simulink model "Sub4"  (R2024a)
settings: Solver=FixedStepDiscrete  StartTime=0.0  StopTime=4.5  FixedStep=75e-6  RelTol=1e-3  EnableMultiTasking=on
undefined symbols (not defined in the file or in its folder): D1, D11, Delta
libraries: spsSeriesRLCBranchLib x41, spsLoadFlowBusLib x29, spsDistributedParametersLineLib x19, spsThreePhaseSeriesRLCLoadLib x15, spsThreePhaseTransformerTwoWindingsLib x13, spsThreePhaseParallelRLCLoadLib x11, spsThreePhaseVIMeasurementLib x11, spsSynchronousMachinepuStandardLib x7, spsExcitationSystemLib x7, spsHydraulicTurbineandGovernorLib x7, spsGenericPowerSystemStabilizerLib x7, spsMultiBandPowerSystemStabilizerLib x7
(part 3 of 5)

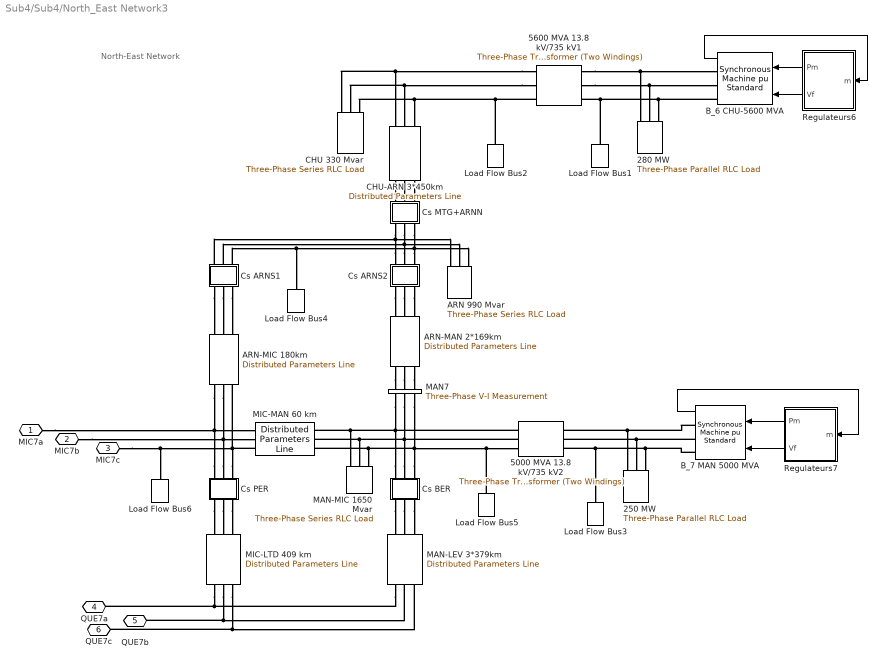
== system Sub4/Sub4/North_East Network3 ==
  note: North-East Network
  250 MW : spsThreePhaseParallelRLCLoadLib/Three-Phase Parallel RLC Load  LConnTagsString=A|B|C  Configuration=Y (grounded)  NominalVoltage=(13800)*1  Vabc=[1e3 1e3 1e3]  Vabcp=[1e3 1e3 1e3]  NominalFrequency=60  UnbalancedPower=off  ActivePower=250000000  InductivePower=0  CapacitivePower=0  Pabc=[10e3 9e3 11e3]  QLabc=[100 90 110]  QCabc=[100 90 110]  Pabcp=[10e3 9e3 11e3]  QLabcp=[100 90 110]  QCabcp=[100 90 110]  Measurements=None  LoadType=constant PQ
  280 MW : spsThreePhaseParallelRLCLoadLib/Three-Phase Parallel RLC Load  LConnTagsString=A|B|C  Configuration=Y (grounded)  NominalVoltage=(13800)*1  Vabc=[1e3 1e3 1e3]  Vabcp=[1e3 1e3 1e3]  NominalFrequency=60  UnbalancedPower=off  ActivePower=280000000  InductivePower=0  CapacitivePower=0  Pabc=[10e3 9e3 11e3]  QLabc=[100 90 110]  QCabc=[100 90 110]  Pabcp=[10e3 9e3 11e3]  QLabcp=[100 90 110]  QCabcp=[100 90 110]  Measurements=None  LoadType=constant PQ
  5000 MVA 13.8 kV/735 kV2 : spsThreePhaseTransformerTwoWindingsLib/Three-Phase Transformer (Two Windings)  Winding1Connection=Delta (D1)  Winding2Connection=Yg  CoreType=Three single-phase transformers  SetSaturation=off  Hysteresis=off  DataFile='basic_model'  SetInitialFlux=off  Measurements=None  UNITS=pu  NominalPower=[ 5000e6 60 ]  Winding1="[ 13.8e3 0.002  0.0]"  Winding2=[ 735e3 0.002 0.12]  Rm=500  Lm=500  L0=0.5  Saturation="[ 0,0  ;  0.005,1.2  ;  1.0,1.4 ]"  InitialFluxes=[ 0.8 , -0.8 , 0.7 ]  BreakLoop=off  DiscreteSolver=Trapezoidal iterative  DataType=off  TransfoNumber=0
  5600 MVA 13.8 kV/735 kV1 : spsThreePhaseTransformerTwoWindingsLib/Three-Phase Transformer (Two Windings)  Winding1Connection=Delta (D1)  Winding2Connection=Yg  CoreType=Three single-phase transformers  SetSaturation=off  Hysteresis=off  DataFile='basic_model'  SetInitialFlux=off  Measurements=None  UNITS=pu  NominalPower=[ 5600e6 60 ]  Winding1="[ 13.8e3 0.002  0.0]"  Winding2=[ 735e3 0.002 0.12]  Rm=500  Lm=500  L0=0.5  Saturation="[ 0,0  ;  0.005,1.2  ;  1.0,1.4 ]"  InitialFluxes=[ 0.8 , -0.8 , 0.7 ]  BreakLoop=off  DiscreteSolver=Trapezoidal iterative  DataType=off  TransfoNumber=0
  ARN 990 Mvar : spsThreePhaseSeriesRLCLoadLib/Three-Phase Series RLC Load  LConnTagsString=A|B|C  Configuration=Y (grounded)  NominalVoltage=735e3  Vabc=[1e3 1e3 1e3]  Vabcp=[1e3 1e3 1e3]  NominalFrequency=60  UnbalancedPower=off  ActivePower=3300000  InductivePower=990e6  CapacitivePower=0  Pabc=[10e3 9e3 11e3]  QLabc=[100 90 110]  QCabc=[100 90 110]  Pabcp=[10e3 9e3 11e3]  QLabcp=[100 90 110]  QCabcp=[100 90 110]  Measurements=None  LoadType=constant Z
  ARN-MAN 2*169km : spsDistributedParametersLineLib/Distributed Parameters Line  Phases=3  Length=169  Frequency=60  Resistance="[0.01273  0.3864]/2"  Inductance="[0.9337e-3  4.1264e-3]/2"  Capacitance=[12.74e-9 7.751e-9]*2  x1=[-0.000975 1.66426565004939e-09 276427.296115043 -784420.047795663;-0.0009 1.59178701377787e-09 298492.841238135 -776291.834335438;-0.000825 1.51803592732269e-09 320319.775751036 -767543.065060509;-0.00075 1.44307134617394e-09 341890.651536257 -758180.733603173;-0.000675 1.36695319587079e-09 363188.225165743 -748212.324067948;-0.0006 1.28974232409794e-09 384195.471684998 -737645.805048896;-0.000525 1.21150045204493e-09 404895.598222576 -726489.623259648;-0.00045 1.13229012506714e-09 425272.057414045 -714752.696781229;-0.000375 1.05217466268798e-09 445308.560629698 -702444.407933087;-0.0003 9.71218107982286e-10 464989.090995432 -689574.595773002;-0.000225 8.89485176381205e-10 484297.916196397 -676153.548231903;-0.00015 8.07041203939704e-10 503219.601053161 -662191.993889842;-7.5e-05 7.23952095107918e-10 521739.019860361 -647701.093399743]  x2=[-0.000975 1.50301647460342e-09 170603.864508789 -782532.609847258;-0.0009 1.45617880236044e-09 192658.333570876 -777396.800423983;-0.000825 1.40817708306313e-09 214558.794508878 -771639.551893019;-0.00075 1.35904968855145e-09 236287.740429409 -765265.466510753;-0.000675 1.3088358905129e-09 257827.801545564 -758279.639623513;-0.0006 1.25757582908933e-09 279161.759062062 -750687.655594424;-0.000525 1.20531048078955e-09 300272.558939683 -742495.583339361;-0.00045 1.15208162573329e-09 321143.325528012 -733709.971475538;-0.000375 1.09793181425286e-09 341757.375055572 -724337.843086658;-0.0003 1.04290433287904e-09 362098.228966576 -714386.690108754;-0.000225 9.87043169738486e-10 382149.627093632 -703864.467341261;-0.00015 9.30392979390309e-10 401895.540655875 -692779.586088062;-7.5e-05 8.72999047129898e-10 421320.185072126 -681140.907433628]  x3=[-0.000975 -6.52958955805801e-13 1329.1720136715 -2414.87241463394;-0.0009 -8.44230426340621e-13 1396.90953145447 -2376.33167069261;-0.000825 -1.03482703198978e-12 1463.53038113142 -2335.89132357282;-0.00075 -1.22459641274296e-12 1528.98130701446 -2293.5837006693;-0.000675 -1.41338686986074e-12 1593.20998863487 -2249.44262204848;-0.0006 -1.6010474871403e-12 1656.1650825673 -2203.50337341321;-0.000525 -1.78742825155548e-12 1717.7962634729 -2155.80267789598;-0.00045 -1.97238017317495e-12 1778.05426432864 -2106.37866670291;-0.000375 -2.1557554042624e-12 1836.89091581062 -2055.27084863236;-0.0003 -2.33740735746385e-12 1894.25918479988 -2002.52007849212;-0.000225 -2.51719082298728e-12 1950.11321197994 -1948.16852444071;-0.00015 -2.69496208468112e-12 2004.40834849608 -1892.25963427884;-7.5e-05 -2.87057903491877e-12 2057.10119164691 -1834.83810071787]  x4=[-0.000975 1.02278224953366e-11 681.724417840483 -9455.17189861565;-0.0009 9.98598605323801e-12 948.756484621656 -9432.11979189438;-0.000825 9.73616696667912e-12 1215.03012998548 -9401.52779292775;-0.00075 9.47856493721543e-12 1480.33249885398 -9363.42035649164;-0.000675 9.21338588796783e-12 1744.45151257275 -9317.8279450877;-0.0006 8.94084179901093e-12 2007.17603844337 -9264.787004592;-0.000525 8.66115053791936e-12 2268.29605849967 -9204.33993512082;-0.00045 8.37453568560783e-12 2527.60283739291 -9136.53505713663;-0.000375 8.08122635760391e-12 2784.88908925156 -9061.42657282144;-0.0003 7.78145702089663e-12 3039.94914338249 -8979.07452274841;-0.000225 7.47546730650714e-12 3292.57910868098 -8889.54473788635;-0.00015 7.1635018179313e-12 3542.57703661814 -8792.90878697541;-7.5e-05 6.84580993560747e-12 3789.74308267548 -8689.24391931618]  x5=0.000955765248222805  V1=ones(3,3)  V2=ones(3,3)  I1=ones(3,3)  I2=ones(3,3)  nHarmo=1  Measurements=None  Decoupling=on  VsMag0=[679080.965035306 679082.342856188 679080.506296934]  VrMag0=[653943.402704951 653944.061381449 653943.214719902]  VsAngle0=[10.4723030523782 -109.527808757273 130.472146471772]  VrAngle0=[3.35889302260268 -116.641159314998 123.358816875039]  IsMag0=[2259.59659727747 2259.62910081935 2259.62302793109]  IrMag0=[7771.00845150682 7771.0004925988 7770.97273571783]  IsAngle0=[19.8888438810371 -100.110858095183 139.888279140977]  IrAngle0=[-4.81594167233342 -124.816211863633 115.183974051701]
      settings: AttributesFormatString=\n  LibrarySourceBlock=sps_lib/Power Grid Elements/Distributed Parameters Line
  ARN-MIC 180km : spsDistributedParametersLineLib/Distributed Parameters Line  Phases=3  Length=180  Frequency=60  Resistance="[0.01273  0.3864]"  Inductance="[0.9337e-3  4.1264e-3]"  Capacitance=[12.74e-9 7.751e-9]  x1=[-0.00105 1.25846980374652e-09 262529.955827328 -774207.772445671;-0.000975 1.18990309098791e-09 284312.34957459 -766476.523484284;-0.0009 1.12038518790449e-09 305867.468379727 -758132.564917507;-0.000825 1.04997166604432e-09 327178.08141057 -749182.566778153;-0.00075 9.78718812899427e-10 348227.153289126 -739633.683557793;-0.000675 9.066835869104e-10 368997.857709397 -729493.548487572;-0.0006 8.33923571934722e-10 389473.590888071 -718770.267436316;-0.000525 7.60496931215097e-10 409637.984837336 -707472.412430826;-0.00045 6.86462360884652e-10 429474.920449193 -695609.014803529;-0.000375 6.11879043046142e-10 448968.540380829 -683189.557972972;-0.0003 5.36806598462684e-10 468103.261730734 -670223.969862923;-0.000225 4.61305038897832e-10 486863.788495431 -656722.614966137;-0.00015 3.85434719143088e-10 505235.123796871 -642696.286059139;-7.5e-05 3.09256288771211e-10 523202.581870704 -628156.195574648]  x2=[-0.00105 4.56021511773203e-09 126759.491965578 -811882.989724351;-0.000975 4.50169247794927e-09 149661.239004126 -807974.954383031;-0.0009 4.43957125407784e-09 172443.349138107 -803421.036225608;-0.000825 4.37390110487363e-09 195087.610697259 -798224.875584581;-0.00075 4.3047345260491e-09 217575.92220536 -792390.626191262;-0.000675 4.23212680830911e-09 239890.306850274 -785922.951855348;-0.0006 4.15613599315226e-09 262012.926854336 -778827.022736746;-0.000525 4.07682282647349e-09 283926.097733603 -771108.511212621;-0.00045 3.99425071000473e-09 305612.302434556 -762773.587342989;-0.000375 3.90848565063247e-09 327054.205336969 -753828.913938461;-0.0003 3.81959620763294e-09 348234.666111732 -744281.641234101;-0.000225 3.7276534378668e-09 369136.753422575 -734139.401173629;-0.00015 3.63273083897744e-09 389743.758460713 -723410.301308568;-7.5e-05 3.53490429063805e-09 410039.208301618 -712102.91831719]  x3=[-0.00105 3.52588969292103e-12 -44.8517351585408 -825.879343626934;-0.000975 3.77869229184614e-12 -21.4861584038212 -826.817643960785;-0.0009 4.02847426196908e-12 1.89659405717708 -827.094998920788;-0.000825 4.27503593140473e-12 25.277830409905 -826.711186793632;-0.00075 4.51818020252705e-12 48.6388600517669 -825.666514392858;-0.000675 4.75771270952595e-12 71.961008533103 -823.9618168136;-0.0006 4.9934419737803e-12 95.2256324852582 -821.598456765019;-0.000525 5.22517955692303e-12 118.414134523806 -818.578323480979;-0.00045 5.45274021147589e-12 141.507978115012 -814.903831209816;-0.000375 5.67594202893342e-12 164.488702393657 -810.577917284431;-0.0003 5.89460658517784e-12 187.337936920371 -805.604039774227;-0.000225 6.10855908310858e-12 210.037416366677 -799.986174720782;-0.00015 6.31762849237237e-12 232.56899511602 -793.728812959465;-7.5e-05 6.52164768608231e-12 254.914661769092 -786.836956529525]  x4=[-0.00105 3.68388905079501e-12 787.856966725056 -5164.02437043881;-0.000975 3.27425714129396e-12 933.532622338121 -5139.68710729563;-0.0009 2.86200784073198e-12 1078.46202625642 -5111.24125691872;-0.000825 2.44747069489231e-12 1222.52932413195 -5078.70955848564;-0.00075 2.03097707842669e-12 1365.61935077109 -5042.11801733838;-0.000675 1.61285992995958e-12 1507.6177221959 -5001.49588419504;-0.0006 1.19345348594203e-12 1648.41092708092 -4956.87563176734;-0.000525 7.73093013468282e-13 1787.88641749236 -4908.29292880234;-0.00045 3.52114542268281e-13 1925.93269885724 -4855.78661156945;-0.000375 -6.91454039092747e-14 2062.43941909041 -4799.39865281531;-0.0003 -4.90350076308906e-13 2197.29745680833 -4739.17412821136;-0.000225 -9.11162770360144e-13 2330.39900855907 -4675.16118032112;-0.00015 -1.33124709483401e-12 2461.63767499866 -4607.41098011569;-7.5e-05 -1.75026724074904e-12 2590.90854594518 -4535.97768606851]  x5=0.00101797482059234  V1=ones(3,3)  V2=ones(3,3)  I1=ones(3,3)  I2=ones(3,3)  nHarmo=1  Measurements=None  Decoupling=on  VsMag0=[667492.500318997 667493.817536454 667492.030186196]  VrMag0=[670930.718084451 670931.402748886 670930.538861588]  VsAngle0=[11.4115363399382 -108.588575536837 131.411382483017]  VrAngle0=[1.55396261635725 -118.446088813397 121.553886266157]  IsMag0=[678.171382863534 678.181184845914 678.186053012205]  IrMag0=[4283.30300695155 4283.29854095558 4283.28683546946]  IsAngle0=[-10.4293295371599 -130.428376510184 109.570429816024]  IrAngle0=[1.35460954054385 -118.645605751902 121.354553630566]
      settings: AttributesFormatString=\n  LibrarySourceBlock=sps_lib/Power Grid Elements/Distributed Parameters Line
  "B_6 CHU-5600 MVA " : spsSynchronousMachinepuStandardLib/Synchronous Machine pu Standard  PresetModel=No  MechanicalLoad=Mechanical power Pm  ShowDetailedParameters=on  RotorType=Salient-pole  Units=per unit standard parameters  MeasurementBus=off  NominalParameters="[ 5600E6  13800   60 ]"  Reactances1=[ 31 32 33 34 35 36 37 ]  Reactances2=[ 1.305, 0.296, 0.252, 0.474, 0.243, 0.18 ]  dAxisTimeConstants=Short-circuit  qAxisTimeConstants=Open-circuit  TimeConstants1=[]  TimeConstants2=[]  TimeConstants3=[]  TimeConstants4=[]  TimeConstants5=[ 1.01, 0.053, 0.1 ]  TimeConstants6=[]  TimeConstants7=[]  TimeConstants8=[]  StatorResistance=2.8544e-3  Mechanical="[ 4.0 0  32]"  PolePairs=32  InitialConditions=[0 -61.7964 0.894782 0.894782 0.894782 8.48442 -111.516 128.484 1.31361]  SetSaturation=off  Saturation=[0.6404,0.7127,0.8441,0.9214,0.9956,1.082,1.19,1.316,1.457;0.7,0.7698,0.8872,0.9466,0.9969,1.046,1.1,1.151,1.201]  LoadFlowParameters=[1 5000000000 0 0 0]  TsPowergui=0  TsBlock=-1  IterativeModel=Trapezoidal non iterative  IterativeDiscreteModel=Trapezoidal non iterative  BusType=PV  Pref=5000000000  Qref=0  Qmin=-Inf  Qmax=Inf  PLF=0  QLF=0
  B_7 MAN 5000 MVA : spsSynchronousMachinepuStandardLib/Synchronous Machine pu Standard  PresetModel=No  MechanicalLoad=Mechanical power Pm  ShowDetailedParameters=on  RotorType=Salient-pole  Units=per unit standard parameters  MeasurementBus=off  NominalParameters="[ 5000E6  13800   60 ]"  Reactances1=[ 31 32 33 34 35 36 37 ]  Reactances2=[ 1.305, 0.296, 0.252, 0.474, 0.243, 0.18 ]  dAxisTimeConstants=Short-circuit  qAxisTimeConstants=Open-circuit  TimeConstants1=[]  TimeConstants2=[]  TimeConstants3=[]  TimeConstants4=[]  TimeConstants5=[ 1.01, 0.053, 0.1 ]  TimeConstants6=[]  TimeConstants7=[]  TimeConstants8=[]  StatorResistance=2.8544e-3  Mechanical="[ 3.7 0  32]"  PolePairs=32  InitialConditions=[0 -81.9543 0.907703 0.907703 0.907703 -8.76021 -128.76 111.24 1.25655]  SetSaturation=off  Saturation=[0.6404,0.7127,0.8441,0.9214,0.9956,1.082,1.19,1.316,1.457;0.7,0.7698,0.8872,0.9466,0.9969,1.046,1.1,1.151,1.201]  LoadFlowParameters=[1 4500000000 0 0 0]  TsPowergui=0  TsBlock=-1  IterativeModel=Trapezoidal non iterative  IterativeDiscreteModel=Trapezoidal non iterative  BusType=PV  Pref=4500000000  Qref=0  Qmin=-Inf  Qmax=Inf  PLF=0  QLF=0
  CHU 330 Mvar : spsThreePhaseSeriesRLCLoadLib/Three-Phase Series RLC Load  LConnTagsString=A|B|C  Configuration=Y (grounded)  NominalVoltage=735e3  Vabc=[1e3 1e3 1e3]  Vabcp=[1e3 1e3 1e3]  NominalFrequency=60  UnbalancedPower=off  ActivePower=1100000  InductivePower=330e6  CapacitivePower=0  Pabc=[10e3 9e3 11e3]  QLabc=[100 90 110]  QCabc=[100 90 110]  Pabcp=[10e3 9e3 11e3]  QLabcp=[100 90 110]  QCabcp=[100 90 110]  Measurements=None  LoadType=constant Z
  CHU-ARN 3*450km : spsDistributedParametersLineLib/Distributed Parameters Line  Phases=3  Length=450  Frequency=60  Resistance="[0.01273  0.3864]/3"  Inductance="[0.9337e-3  4.1264e-3]/3"  Capacitance=[12.74e-9 7.751e-9]*3  x1=[-0.00255 1.83974130674967e-09 0 0;-0.002475 1.75252338019027e-09 0 0;-0.0024 1.66390451325524e-09 0 0;-0.002325 1.57395554651092e-09 0 0;-0.00225 1.48274838378504e-09 0 0;-0.002175 1.39035593468798e-09 0 0;-0.0021 1.29685205632988e-09 0 0;-0.002025 1.20231149428046e-09 0 0;-0.00195 1.10680982281849e-09 0 0;-0.001875 1.01042338451892e-09 0 0;-0.0018 9.13229229225756e-10 0 0;-0.001725 8.15305052459629e-10 0 0;-0.00165 7.1672913330915e-10 0 0;-0.001575 6.17580271855829e-10 242668.42145696 -732167.508894537;-0.0015 5.17937726182481e-10 263270.288908628 -725014.590467308;-0.001425 4.17881149015535e-10 283661.702119514 -717282.106469554;-0.00135 3.17490524051862e-10 303826.360505894 -708976.238130673;-0.001275 2.1684610202103e-10 323748.144748385 -700103.62503473;-0.0012 1.160283365341e-10 343411.129677477 -690671.359812879;-0.001125 1.51178197702368e-11 362799.597003872 -680686.98247362;-0.00105 -8.58047819474405e-11 381898.047883441 -670158.474375432;-0.000975 -1.86658792635286e-10 400691.215306768 -659094.251846596;-0.0009 -2.87363591140274e-10 419164.076303361 -647503.159457315;-0.000825 -3.87838675587315e-10 437301.863950782 -635394.462949494;-0.00075 -4.88003727731222e-10 455090.079179103 -622777.841829852;-0.000675 -5.87778677161888e-10 472514.502361241 -609663.381632272;-0.0006 -6.87083765311346e-10 489561.204679905 -596061.565855578;-0.000525 -7.85839609211549e-10 506216.559262086 -581983.267583187;-0.00045 -8.83967264951897e-10 522467.252072166 -567439.740791332;-0.000375 -9.81388290785795e-10 538300.292554956 -552442.611352808;-0.0003 -1.07802480983578e-09 553703.024020149 -537003.867743423;-0.000225 -1.17379957234712e-09 568663.13375988 -521135.8514586;-0.00015 -1.26863601744006e-09 583168.662891321 -504851.247147766;-7.5e-05 -1.36245833431144e-09 597208.015916427 -488163.072474445]  x2=[-0.00255 2.68580757791396e-09 0 0;-0.002475 2.65982228221435e-09 0 0;-0.0024 2.63171076527898e-09 0 0;-0.002325 2.60149549902437e-09 0 0;-0.00225 2.56920063707206e-09 0 0;-0.002175 2.53485199544056e-09 0 0;-0.0021 2.49847703190844e-09 0 0;-0.002025 2.460104824065e-09 0 0;-0.00195 2.41976604606606e-09 0 0;-0.001875 2.37749294411356e-09 0 0;-0.0018 2.3333193106784e-09 0 0;-0.001725 2.28728045748726e-09 0 0;-0.00165 2.23941318729497e-09 0 0;-0.001575 2.18975576446493e-09 -54170.285736792 -807523.190587312;-0.0015 2.13834788438116e-09 -31319.4766467201 -808731.868853913;-0.001425 2.08523064171644e-09 -8443.63124622096 -809294.059238565;-0.00135 2.03044649758183e-09 14438.9638639046 -809209.312334876;-0.001275 1.97403924558393e-09 37310.0166872409 -808477.695888224;-0.0012 1.91605397681692e-09 60151.2444540997 -807099.794741603;-0.001125 1.85653704381745e-09 82944.3882364869 -805076.710368106;-0.00105 1.79553602351112e-09 105671.227544009 -802410.059990428;-0.000975 1.73309967918022e-09 128313.594889057 -799101.975288079;-0.0009 1.66927792148309e-09 150853.390309615 -795155.100693355;-0.000825 1.60412176855635e-09 173272.595838093 -790572.591277418;-0.00075 1.5376833052317e-09 195553.289904618 -785358.11022818;-0.000675 1.4700156414002e-09 217677.661663259 -779515.825922007;-0.0006 1.40117286955695e-09 239628.025229746 -773050.408591585;-0.000525 1.33121002156044e-09 261386.833819296 -765967.026592602;-0.00045 1.2601830246409e-09 282936.693773244 -758271.342272249;-0.000375 1.1881486566929e-09 304260.378463266 -749969.507442825;-0.0003 1.11516450088803e-09 325340.842062084 -741068.158464069;-0.000225 1.04128889964374e-09 346161.23316964 -731574.410938161;-0.00015 9.66580907985323e-10 366704.908283844 -721495.854021612;-7.5e-05 8.91100246338249e-10 386955.44510514 -710840.544358615]  x3=[-0.00255 5.22946667910045e-12 0 0;-0.002475 5.11024941511311e-12 0 0;-0.0024 4.98694709593276e-12 0 0;-0.002325 4.85965828754678e-12 0 0;-0.00225 4.728484742681e-12 0 0;-0.002175 4.59353131946016e-12 0 0;-0.0021 4.45490589758593e-12 0 0;-0.002025 4.31271929209951e-12 0 0;-0.00195 4.16708516479781e-12 0 0;-0.001875 4.01811993337391e-12 0 0;-0.0018 3.86594267835457e-12 0 0;-0.001725 3.71067504790906e-12 0 0;-0.00165 3.55244116060548e-12 0 0;-0.001575 3.39136750619228e-12 -1464.09976005102 -2947.40439175083;-0.0015 3.2275828444843e-12 -1380.19037065383 -2987.61903902528;-0.001425 3.06121810243411e-12 -1295.17767819195 -3025.44542935204;-0.00135 2.89240626947105e-12 -1209.12964051102 -3060.85332489344;-0.001275 2.72128229119146e-12 -1122.11504309576 -3093.81442111955;-0.0012 2.54798296148532e-12 -1034.20344408399 -3124.30236943436;-0.001125 2.37264681318521e-12 -945.465118662861 -3152.29279823848;-0.00105 2.19541400732535e-12 -855.971002891975 -3177.76333241138;-0.000975 2.016426221099e-12 -765.792636998172 -3200.69361119776;-0.0009 1.83582653460386e-12 -675.002108187373 -3221.06530448361;-0.000825 1.65375931646604e-12 -583.671993019167 -3238.862127449;-0.00075 1.47037010843401e-12 -491.875299390224 -3254.06985358596;-0.000675 1.28580550903471e-12 -399.685408172891 -3266.67632607091;-0.0006 1.10021305638497e-12 -307.176014555658 -3276.67146748261;-0.000525 9.13741110251785e-13 -214.421069132339 -3284.04728785797;-0.00045 7.26538733455771e-13 -121.494718787109 -3288.79789107902;-0.000375 5.38755572712647e-13 -28.471247422611 -3290.91947958624;-0.0003 3.50541739007934e-13 64.5749834214516 -3290.41035741423;-0.000225 1.62047687600526e-13 157.569594011797 -3287.27093154747;-0.00015 -2.65759022489375e-14 250.438245879586 -3281.50371159497;-7.5e-05 -2.15178247728768e-13 343.106701245452 -3273.1133077841]  x4=[-0.00255 2.03747390835008e-11 0 0;-0.002475 2.02149529085469e-11 0 0;-0.0024 2.00390072095371e-11 0 0;-0.002325 1.9847042634771e-11 0 0;-0.00225 1.96392126377927e-11 0 0;-0.002175 1.94156833547217e-11 0 0;-0.0021 1.91766334714469e-11 0 0;-0.002025 1.89222540807874e-11 0 0;-0.00195 1.86527485297358e-11 0 0;-0.001875 1.83683322569062e-11 0 0;-0.0018 1.80692326203154e-11 0 0;-0.001725 1.77556887156364e-11 0 0;-0.00165 1.74279511850693e-11 0 0;-0.001575 1.70862820169814e-11 -1565.83540459129 -14460.8260986656;-0.0015 1.6730954336478e-11 -1156.39187005829 -14499.3124213137;-0.001425 1.63622521870703e-11 -746.02393355776 -14526.2082154592;-0.00135 1.5980470303615e-11 -335.05963693929 -14541.4919810156;-0.001275 1.55859138767084e-11 76.172501226366 -14545.1515003748;-0.0012 1.51788983087213e-11 487.34374826002 -14537.1838481728;-0.001125 1.47597489616711e-11 898.125420157924 -14517.595393629;-0.00105 1.43288008971327e-11 1308.18914433673 -14486.4017954541;-0.000975 1.38863986083951e-11 1717.20712212953 -14443.6279893333;-0.0009 1.3432895745079e-11 2124.85239082304 -14389.3081679928;-0.000825 1.29686548304345e-11 2530.79908502666 -14323.4857538666;-0.00075 1.24940469715455e-11 2934.72269716423 -14246.2133643855;-0.000675 1.20094515626729e-11 3336.30033688045 -14157.5527699152;-0.0006 1.15152559819719e-11 3735.21098915448 -14057.5748443784;-0.000525 1.10118552818281e-11 4131.13577091443 -13946.3595085992;-0.00045 1.04996518730591e-11 4523.7581859476 -13823.9956664153;-0.000375 9.9790552032329e-12 4912.76437790274 -13690.5811336098;-0.0003 9.45048142936186e-12 5297.84338118201 -13546.2225597191;-0.000225 8.9143530852334e-12 5678.68736952208 -13391.0353427783;-0.00015 8.37109874364277e-12 6054.99190206578 -13225.1435370742;-7.5e-05 7.82115267379859e-12 6426.45616672746 -13048.679753978]  x5=0.00254493705148084  V1=ones(3,3)  V2=ones(3,3)  I1=ones(3,3)  I2=ones(3,3)  nHarmo=1  Measurements=None  Decoupling=on  VsMag0=[629792.48162364 629794.239253206 629791.265031655]  VrMag0=[660822.00206013 660822.394547621 660821.800733162]  VsAngle0=[22.3571846561267 -97.6430354653443 142.356936116218]  VrAngle0=[0.182246528172093 -119.817793275379 120.182197155401]  IsMag0=[2715.66118101666 2715.69463660214 2715.70679003246]  IrMag0=[12002.6021032761 12002.5859963174 12002.5499905605]  IsAngle0=[-22.3962421231331 -142.395538519995 97.6034984022445]  IrAngle0=[-2.15980439262474 -122.160047251323 117.840140765696]
      settings: AttributesFormatString=\n  LibrarySourceBlock=sps_lib/Power Grid Elements/Distributed Parameters Line
  "Cs ARNS1 " : Subsystem  mask{Xc=25}
      mask prompts: Xc "Condensator Reactance at  60Hz  (ohm):"
      mask help: Series Compensation
      mask init:
      | Cs=1/Xc/(2*pi*60);
      mask Display: disp('Cs')
  Cs ARNS2 : Subsystem  mask{Xc=25/2}
      mask prompts: Xc "Condensator Reactance at  60Hz  (ohm):"
      mask help: Series Compensation
      mask init:
      | Cs=1/Xc/(2*pi*60);
      mask Display: disp('Cs')
  Cs BER : Subsystem  mask{Xc=22/3}
      mask prompts: Xc "Condensator Reactance at  60Hz  (ohm):"
      mask help: Series Compensation
      mask init:
      | Cs=1/Xc/(2*pi*60);
      mask Display: disp('Cs')
  "Cs MTG+ARNN " : Subsystem  mask{Xc=(30+25)/3}
      mask prompts: Xc "Condensator Reactance at  60Hz  (ohm):"
      mask help: Series Compensation
      mask init:
      | Cs=1/Xc/(2*pi*60);
      mask Display: disp('Cs')
  "Cs PER " : Subsystem  mask{Xc=22}
      mask prompts: Xc "Condensator Reactance at  60Hz  (ohm):"
      mask help: Series Compensation
      mask init:
      | Cs=1/Xc/(2*pi*60);
      mask Display: disp('Cs')
  Load Flow Bus1 : spsLoadFlowBusLib/Load Flow Bus  LConnTagsString=a  Phases=single  Connectors=on one side  ID=CHU_13.8  Vbase=13.8e3  Vref=1  Vangle=0  VLF=1  VLFb=1  VLFc=1  angleLF=4.726  angleLFb=0  angleLFc=0
      settings: AttributesFormatString=%<ID>\n%<Vbase>V\n%<VLF>pu\n%<angleLF>deg.
  Load Flow Bus2 : spsLoadFlowBusLib/Load Flow Bus  LConnTagsString=a  Phases=single  Connectors=on one side  ID=CHU7  Vbase=735e3  Vref=1  Vangle=0  VLF=1.009  VLFb=1  VLFc=1  angleLF=28.97  angleLFb=0  angleLFc=0
      settings: AttributesFormatString=%<ID>\n%<Vbase>V\n%<VLF>pu\n%<angleLF>deg.
  Load Flow Bus3 : spsLoadFlowBusLib/Load Flow Bus  LConnTagsString=a  Phases=single  Connectors=on one side  ID=MAN_13.8  Vbase=13.8e3  Vref=1  Vangle=0  VLF=1  VLFb=1  VLFc=1  angleLF=-16.23  angleLFb=0  angleLFc=0
      settings: AttributesFormatString=%<ID>\n%<Vbase>V\n%<VLF>pu\n%<angleLF>deg.
  Load Flow Bus4 : spsLoadFlowBusLib/Load Flow Bus  LConnTagsString=a  Phases=single  Connectors=on one side  ID=ARN7  Vbase=735e3  Vref=1  Vangle=0  VLF=1.054  VLFb=1  VLFc=1  angleLF=12.72  angleLFb=0  angleLFc=0
      settings: AttributesFormatString=%<ID>\n%<Vbase>V\n%<VLF>pu\n%<angleLF>deg.
  Load Flow Bus5 : spsLoadFlowBusLib/Load Flow Bus  LConnTagsString=a  Phases=single  Connectors=on one side  ID=MAN7  Vbase=735e3  Vref=1  Vangle=0  VLF=1.016  VLFb=1  VLFc=1  angleLF=7.996  angleLFb=0  angleLFc=0
      settings: AttributesFormatString=%<ID>\n%<Vbase>V\n%<VLF>pu\n%<angleLF>deg.
  Load Flow Bus6 : spsLoadFlowBusLib/Load Flow Bus  LConnTagsString=a  Phases=single  Connectors=on one side  ID=MIC7  Vbase=735e3  Vref=1  Vangle=0  VLF=1.041  VLFb=1  VLFc=1  angleLF=5.981  angleLFb=0  angleLFc=0
      settings: AttributesFormatString=%<ID>\n%<Vbase>V\n%<VLF>pu\n%<angleLF>deg.
  MAN-LEV 3*379km : spsDistributedParametersLineLib/Distributed Parameters Line  Phases=3  Length=379  Frequency=60  Resistance="[0.01273  0.3864]/3"  Inductance="[0.9337e-3  4.1264e-3]/3"  Capacitance=[12.74e-9 7.751e-9]*3  x1=[-0.002175 3.15897921538655e-09 -129715.856576167 -778750.814673074;-0.0021 3.11714336209132e-09 -107648.251269329 -782106.718665579;-0.002025 3.07281571208632e-09 -85494.5935974998 -784837.418513817;-0.00195 3.02603170021674e-09 -63272.5928556595 -786940.73133811;-0.001875 2.97682872490585e-09 -41000.0129711937 -788414.975782369;-0.0018 2.92524611825927e-09 -18694.6583036801 -789258.97335814;-0.001725 2.87132511462352e-09 3625.64058764389 -789472.049386677;-0.00165 2.81510881762389e-09 25943.0411973561 -789054.033538261;-0.001575 2.75664216570806e-09 48239.7033368772 -788005.259968366;-0.0015 2.695971896223e-09 70497.8033956427 -786326.567050537;-0.001425 2.63314650805386e-09 92699.5485890265 -784019.296706208;-0.00135 2.56821622285467e-09 114827.191181619 -781085.293331989;-0.001275 2.50123294490195e-09 136863.042674496 -777526.902325287;-0.0012 2.43225021960323e-09 158789.487945133 -773346.968209426;-0.001125 2.36132319069363e-09 180588.999328668 -768548.832359784;-0.00105 2.28850855615485e-09 202244.150629244 -763136.330332746;-0.000975 2.21386452289164e-09 223737.631050246 -757113.788799616;-0.0009 2.13745076020208e-09 245052.259032287 -750486.02208795;-0.000825 2.05932835207892e-09 266170.995987883 -743258.328333047;-0.00075 1.97955974837988e-09 287076.959921839 -735436.485242709;-0.000675 1.89820871490627e-09 307753.438926458 -727026.745478624;-0.0006 1.81534028242953e-09 328183.904540785 -718035.831658085;-0.000525 1.73102069470666e-09 348352.024963204 -708470.930980035;-0.00045 1.64531735552594e-09 368241.678106832 -698339.689479729;-0.000375 1.55829877482541e-09 387836.964487269 -687650.205916608;-0.0003 1.47003451392706e-09 407122.219932398 -676411.025300278;-0.000225 1.38059512993055e-09 426082.028104093 -664631.132059759;-0.00015 1.290052119311e-09 444701.232821795 -652319.942861469;-7.5e-05 1.19847786076572e-09 462964.950178136 -639487.299081685]  x2=[-0.002175 1.41372964042643e-08 -453830.168532102 -672756.853007419;-0.0021 1.420658784343e-08 -434629.546160143 -685317.991887277;-0.002025 1.42645227536416e-08 -415081.487579038 -697331.298050137;-0.00195 1.43110548226185e-08 -395201.619207723 -708787.168242863;-0.001875 1.43461468533367e-08 -375005.832708801 -719676.444818102;-0.0018 1.43697707937638e-08 -354510.272284993 -729990.423054773;-0.001725 1.43819077592831e-08 -333731.321773709 -739720.858116482;-0.00165 1.43825480477903e-08 -312685.59155006 -748859.971642321;-0.001575 1.43716911474484e-08 -291389.905248775 -757400.457964771;-0.0015 1.43493457370976e-08 -269861.28631565 -765335.48994974;-0.001425 1.43155296793168e-08 -248116.94439926 -772658.724454069;-0.00135 1.42702700061453e-08 -226174.261593834 -779364.307396144;-0.001275 1.42136028974734e-08 -204050.778544272 -785446.87843556;-0.0012 1.41455736521206e-08 -181764.180424424 -790901.575258095;-0.001125 1.40662366516249e-08 -159332.282799829 -795724.037462569;-0.00105 1.39756553167705e-08 -136773.01738623 -799910.410046481;-0.000975 1.38739020568906e-08 -114104.41771523 -803457.346487641;-0.0009 1.37610582119842e-08 -91344.6047185641 -806362.011419329;-0.000825 1.36372139876944e-08 -68511.7722425057 -808622.082896841;-0.00075 1.35024683831992e-08 -45624.1725039819 -810235.754253618;-0.000675 1.33569291120732e-08 -22700.1015000316 -811201.735545468;-0.0006 1.32007125161829e-08 242.115617734555 -811519.254581725;-0.000525 1.30339434726848e-08 23184.1391919804 -811188.05754253;-0.00045 1.28567552942006e-08 46107.6297200854 -810208.40918173;-0.000375 1.26692896222492e-08 68994.2625144626 -808581.092615234;-0.0003 1.24716963140205e-08 91825.7423510333 -806307.408695007;-0.000225 1.22641333225816e-08 114583.81809415 -803389.174969186;-0.00015 1.20467665706122e-08 137250.297286273 -799828.724229161;-7.5e-05 1.1819769817768e-08 159807.060690745 -795628.902644777]  x3=[-0.002175 3.97516669926384e-12 -1369.21748804203 -554.792265214498;-0.0021 5.58630848605986e-12 -1352.98611910222 -593.279680635689;-0.002025 7.19298466332552e-12 -1335.67319376017 -631.292837357663;-0.00195 8.79391087870767e-12 -1317.29255170352 -668.801348244557;-0.001875 1.03878073762847e-11 -1297.85888613629 -705.775229566668;-0.0018 1.1973400019584e-11 -1277.38773203339 -742.184924968987;-0.001725 1.35494213101067e-11 -1255.89545372219 -778.001329098096;-0.00165 1.51146114005473e-11 -1233.39923180113 -813.195810868544;-0.001575 1.66677191018955e-11 -1209.91704940581 -847.740236350096;-0.0015 1.82075028836184e-11 -1185.46767783355 -881.606991257571;-0.001425 1.97327318661202e-11 -1160.07066153789 -914.769003025273;-0.00135 2.12421868046892e-11 -1133.74630250507 -947.199762448392;-0.001275 2.27346610641428e-11 -1106.51564402493 -978.873344874053;-0.0012 2.42089615833938e-11 -1078.40045386921 -1009.76443092509;-0.001125 2.56639098291645e-11 -1049.42320689075 -1039.84832673995;-0.00105 2.70983427380888e-11 -1019.60706705742 -1069.10098371263;-0.000975 2.85111136464468e-11 -988.97586893519 -1097.49901771673;-0.0009 2.99010932067906e-11 -957.554098635172 -1125.01972779836;-0.000825 3.12671702907268e-11 -925.366874239774 -1151.64111432297;-0.00075 3.26082528771364e-11 -892.439925723698 -1177.34189656148;-0.000675 3.3923268925119e-11 -858.799574385786 -1202.10152970183;-0.0006 3.52111672309663e-11 -824.472711808184 -1225.90022127209;-0.000525 3.64709182684781e-11 -789.486778359619 -1248.71894696238;-0.00045 3.77015150119499e-11 -753.869741259986 -1270.53946583251;-0.000375 3.89019737411736e-11 -717.650072223783 -1291.34433489355;-0.0003 4.00713348278087e-11 -680.856724700259 -1311.11692305151;-0.000225 4.12086635024945e-11 -643.519110728467 -1329.84142440195;-0.00015 4.23130506020901e-11 -605.667077425731 -1347.50287086497;-7.5e-05 4.33836132964458e-11 -567.330883128317 -1364.08714415051]  x4=[-0.002175 5.40742034254097e-11 -9019.35016941118 -13700.3757737279;-0.0021 5.32621970198623e-11 -8628.42708034803 -13949.8814959047;-0.002025 5.24076136289563e-11 -8230.6065586962 -14188.2358962539;-0.00195 5.15111363935786e-11 -7826.20661609385 -14415.248437915;-0.001875 5.05734819439147e-11 -7415.55052366758 -14630.7376505355;-0.0018 4.9595399826585e-11 -6998.96655361441 -14834.5312753359;-0.001725 4.85776719054691e-11 -6576.78771678606 -15026.4664028108;-0.00165 4.75211117366952e-11 -6149.35149648515 -15206.3896029559;-0.001575 4.64265639182964e-11 -5716.99957868617 -15374.157047918;-0.0015 4.52949034150516e-11 -5280.07757889702 -15529.6346269685;-0.001425 4.4127034859052e-11 -4838.93476587919 -15672.6980537095;-0.00135 4.29238918265524e-11 -4393.92378244771 -15803.2329654267;-0.001275 4.16864360916842e-11 -3945.40036357382 -15921.135014509;-0.0012 4.04156568576281e-11 -3493.72305201595 -16026.3099518622;-0.001125 3.91125699658604e-11 -3039.25291170605 -16118.6737022506;-0.00105 3.77782170841044e-11 -2582.35323912066 -16198.1524315054;-0.000975 3.64136648736374e-11 -2123.38927286724 -16264.6826055466;-0.0009 3.50200041366182e-11 -1662.72790171804 -16318.2110411708;-0.000825 3.35983489441162e-11 -1200.7373713248 -16358.6949485657;-0.00075 3.21498357455402e-11 -737.786989848818 -16386.1019655152;-0.000675 3.06756224601783e-11 -274.24683274167 -16400.4101832692;-0.0006 2.91768875515744e-11 189.512553087454 -16401.6081640574;-0.000525 2.76548290854832e-11 653.120445481279 -16389.6949502322;-0.00045 2.61106637721541e-11 1116.20624338406 -16364.6800650346;-0.000375 2.45456259937121e-11 1578.39976309442 -16326.583504981;-0.0003 2.29609668174114e-11 2039.33153418448 -16275.4357238787;-0.000225 2.13579529955515e-11 2498.63309484893 -16211.2776084811;-0.00015 1.97378659528545e-11 2955.93728644773 -16134.1604458043;-7.5e-05 1.81020007621143e-11 3410.8785470071 -16044.1458821279]  x5=0.00214340253891386  V1=ones(3,3)  V2=ones(3,3)  I1=ones(3,3)  I2=ones(3,3)  nHarmo=1  Measurements=None  Decoupling=on  VsMag0=[644608.259457177 644608.981755895 644608.022803535]  VrMag0=[662602.894278686 662603.037872394 662602.72616328]  VsAngle0=[7.52314012710057 -112.47692122849 127.523053849338]  VrAngle0=[-17.0228975012844 -137.022921456005 102.977079768211]  IsMag0=[1217.0465646787 1217.0479082792 1217.06108392243]  IrMag0=[13512.6448948106 13512.6449098294 13512.625660391]  IsAngle0=[-50.9633701968443 -170.962617439554 69.0369514033924]  IrAngle0=[-16.3779589453629 -136.378053156044 103.621993894147]
      settings: AttributesFormatString=\n  LibrarySourceBlock=sps_lib/Power Grid Elements/Distributed Parameters Line
  MAN-MIC 1650 Mvar : spsThreePhaseSeriesRLCLoadLib/Three-Phase Series RLC Load  LConnTagsString=A|B|C  Configuration=Y (grounded)  NominalVoltage=735e3  Vabc=[1e3 1e3 1e3]  Vabcp=[1e3 1e3 1e3]  NominalFrequency=60  UnbalancedPower=off  ActivePower=5500000  InductivePower=1650e6  CapacitivePower=0  Pabc=[10e3 9e3 11e3]  QLabc=[100 90 110]  QCabc=[100 90 110]  Pabcp=[10e3 9e3 11e3]  QLabcp=[100 90 110]  QCabcp=[100 90 110]  Measurements=None  LoadType=constant Z
  MAN7 : spsThreePhaseVIMeasurementLib/Three-Phase V-I Measurement  VoltageMeasurement=no  SetLabelV=on  LabelV=Vabc_MAN7  Vpu=on  VpuLL=off  CurrentMeasurement=no  SetLabelI=on  LabelI=Iabc_MAN7  Ipu=on  Pbase=100e6  Vbase=735e3  OutputType=Magnitude  PhasorSimulation=off  PSBequivalent=0
  MIC-LTD 409 km : spsDistributedParametersLineLib/Distributed Parameters Line  Phases=3  Length=409  Frequency=60  Resistance="[0.01273  0.3864]"  Inductance="[0.9337e-3  4.1264e-3]"  Capacitance=[12.74e-9 7.751e-9]  x1=[-0.002325 4.73228012673005e-09 0 0;-0.00225 4.74319529559715e-09 0 0;-0.002175 4.75031882671827e-09 0 0;-0.0021 4.75364502565162e-09 0 0;-0.002025 4.75317123348468e-09 0 0;-0.00195 4.74889782895964e-09 0 0;-0.001875 4.74082822817071e-09 0 0;-0.0018 4.72896888183329e-09 0 0;-0.001725 4.71332927012738e-09 0 0;-0.00165 4.69392189511928e-09 0 0;-0.001575 4.67076227076764e-09 0 0;-0.0015 4.6438689105218e-09 0 0;-0.001425 4.61326331252247e-09 59193.0163102158 -807702.943453962;-0.00135 4.57896994241641e-09 82003.602334171 -805706.722469148;-0.001275 4.54101621379897e-09 104748.635933117 -803066.431858118;-0.0012 4.4994324663001e-09 127409.935075207 -799784.182228789;-0.001125 4.45425194133129e-09 149969.384664634 -795862.597361294;-0.00105 4.40551075551292e-09 172408.95102257 -791304.812110575;-0.000975 4.35324787180317e-09 194710.696303003 -786114.469900425;-0.0009 4.29750506835162e-09 216856.792831985 -780295.719810991;-0.000825 4.23832690510247e-09 238829.537358798 -773853.213262065;-0.00075 4.17576068817396e-09 260611.36520766 -766792.100294808;-0.000675 4.1098564320426e-09 282184.864318663 -759118.025454888;-0.0006 4.04066681956237e-09 303532.789166703 -750837.123280315;-0.000525 3.96824715985087e-09 324638.07454729 -741956.013397585;-0.00045 3.89265534407599e-09 345483.849218214 -732481.795230052;-0.000375 3.81395179917869e-09 366053.449386152 -722422.04232276;-0.0003 3.73219943956854e-09 386330.432027457 -711784.796288263;-0.000225 3.64746361683097e-09 406298.588032453 -700578.560378286;-0.00015 3.55981206748617e-09 425941.955162752 -688812.292686354;-7.5e-05 3.46931485884157e-09 445244.830811225 -676495.398986829]  x2=[-0.002325 1.39648745350935e-08 0 0;-0.00225 1.4056703826661e-08 0 0;-0.002175 1.41372964042643e-08 0 0;-0.0021 1.420658784343e-08 0 0;-0.002025 1.42645227536416e-08 0 0;-0.00195 1.43110548226185e-08 0 0;-0.001875 1.43461468533367e-08 0 0;-0.0018 1.43697707937638e-08 0 0;-0.001725 1.43819077592831e-08 0 0;-0.00165 1.43825480477903e-08 0 0;-0.001575 1.43716911474484e-08 0 0;-0.0015 1.43493457370976e-08 0 0;-0.001425 1.43155296793168e-08 -248116.94439926 -772658.724454069;-0.00135 1.42702700061453e-08 -226174.261593834 -779364.307396144;-0.001275 1.42136028974734e-08 -204050.778544272 -785446.87843556;-0.0012 1.41455736521206e-08 -181764.180424424 -790901.575258095;-0.001125 1.40662366516249e-08 -159332.282799829 -795724.037462569;-0.00105 1.39756553167705e-08 -136773.01738623 -799910.410046481;-0.000975 1.38739020568906e-08 -114104.41771523 -803457.346487641;-0.0009 1.37610582119842e-08 -91344.6047185641 -806362.011419329;-0.000825 1.36372139876944e-08 -68511.7722425057 -808622.082896841;-0.00075 1.35024683831992e-08 -45624.1725039819 -810235.754253618;-0.000675 1.33569291120732e-08 -22700.1015000316 -811201.735545468;-0.0006 1.32007125161829e-08 242.115617734555 -811519.254581725;-0.000525 1.30339434726848e-08 23184.1391919804 -811188.05754253;-0.00045 1.28567552942006e-08 46107.6297200854 -810208.40918173;-0.000375 1.26692896222492e-08 68994.2625144626 -808581.092615234;-0.0003 1.24716963140205e-08 91825.7423510333 -806307.408695007;-0.000225 1.22641333225816e-08 114583.81809415 -803389.174969186;-0.00015 1.20467665706122e-08 137250.297286273 -799828.724229161;-7.5e-05 1.1819769817768e-08 159807.060690745 -795628.902644777]  x3=[-0.002325 3.26340431656571e-12 0 0;-0.00225 3.78755932645928e-12 0 0;-0.002175 4.30868661937889e-12 0 0;-0.0021 4.82636961414008e-12 0 0;-0.002025 5.34019448287766e-12 0 0;-0.00195 5.84975048185334e-12 0 0;-0.001875 6.35463027979802e-12 0 0;-0.0018 6.85443028352612e-12 0 0;-0.001725 7.34875096056188e-12 0 0;-0.00165 7.83719715851942e-12 0 0;-0.001575 8.31937842098158e-12 0 0;-0.0015 8.79490929962476e-12 0 0;-0.001425 9.26340966234046e-12 -412.085781584572 -775.710829515535;-0.00135 9.72450499710699e-12 -389.991383899643 -787.050857738754;-0.001275 1.01778267113688e-11 -367.585233069492 -797.761729548578;-0.0012 1.06230124266834e-11 -344.885240228269 -807.834882837965;-0.001125 1.10597062684017e-11 -321.909551402928 -817.262265282299;-0.00105 1.14875591501483e-11 -298.676533007576 -826.036340776299;-0.000975 1.19062290528757e-11 -275.204757161643 -834.150095458262;-0.0009 1.23153812982697e-11 -251.512986843609 -841.59704331684;-0.000825 1.27146888162856e-11 -227.62016089217 -848.371231375857;-0.00075 1.31038324066029e-11 -203.545378866818 -854.467244453027;-0.000675 1.34825009937898e-11 -179.30788577995 -859.880209488769;-0.0006 1.38503918759714e-11 -154.927056712691 -864.605799441654;-0.000525 1.42072109668054e-11 -130.42238132676 -868.640236747377;-0.00045 1.45526730305702e-11 -105.813448284725 -871.980296338486;-0.000375 1.48865019101778e-11 -81.1199295911322 -874.623308222448;-0.0003 1.52084307479294e-11 -56.3615648670004 -876.567159616003;-0.000225 1.5518202198838e-11 -31.5581455702748 -877.810296634087;-0.00015 1.58155686363453e-11 -6.72949917483606 -878.351725531991;-7.5e-05 1.61002923502709e-11 18.1045266792782 -878.191013499736]  x4=[-0.002325 1.59746416946561e-11 0 0;-0.00225 1.58774424359353e-11 0 0;-0.002175 1.57675509926643e-11 0 0;-0.0021 1.56450552103814e-11 0 0;-0.002025 1.55100530103406e-11 0 0;-0.00195 1.53626523112352e-11 0 0;-0.001875 1.52029709429286e-11 0 0;-0.0018 1.50311365522635e-11 0 0;-0.001725 1.48472865010226e-11 0 0;-0.00165 1.46515677561239e-11 0 0;-0.001575 1.44441367721375e-11 0 0;-0.0015 1.42251593662181e-11 0 0;-0.001425 1.39948105855536e-11 -1850.18013712951 -4788.09574636309;-0.00135 1.37532745674348e-11 -1714.07818949525 -4838.48753312546;-0.001275 1.35007443920589e-11 -1576.60603398259 -4885.0115069852;-0.0012 1.32374219281844e-11 -1437.87356372924 -4927.63047738944;-0.001125 1.29635176717598e-11 -1297.99167934925 -4966.31037538532;-0.00105 1.26792505776569e-11 -1157.07220028073 -5001.02028085422;-0.000975 1.23848478846412e-11 -1015.22777539911 -5031.73244722878;-0.0009 1.20805449337211e-11 -872.57179296733 -5058.42232367311;-0.000825 1.17665849800195e-11 -729.218289995053 -5081.06857470836;-0.00075 1.14432189983196e-11 -585.281861079167 -5099.65309726794;-0.000675 1.11107054824396e-11 -440.877566798647 -5114.16103516887;-0.0006 1.07693102385965e-11 -296.120841736882 -5124.58079098758;-0.000525 1.04193061729246e-11 -151.127402205033 -5130.90403533069;-0.00045 1.00609730733188e-11 -6.01315374018816 -5133.12571349341;-0.000375 9.6945973857762e-12 139.105901547752 -5131.24404950023;-0.0003 9.32047198541575e-12 284.113757706387 -5125.26054752455;-0.000225 8.93889594235816e-12 428.894497674198 -5115.17999068629;-0.00015 8.55017428265395e-12 573.332385942874 -5101.01043722835;-7.5e-05 8.15461774445023e-12 717.311961074506 -5082.76321407497]  x5=0.00231306500901259  V1=ones(3,3)  V2=ones(3,3)  I1=ones(3,3)  I2=ones(3,3)  nHarmo=1  Measurements=None  Decoupling=on  VsMag0=[661255.450009799 661256.198077723 661255.233015368]  VrMag0=[662602.894278686 662603.037872394 662602.72616328]  VsAngle0=[4.97147028274463 -115.028588850405 124.971384582259]  VrAngle0=[-17.0228975012844 -137.022921456005 102.977079768211]  IsMag0=[724.117205145966 724.119993409295 724.122226064492]  IrMag0=[4231.68630935734 4231.68661611235 4231.68036878114]  IsAngle0=[-27.1991957967962 -147.198864433647 92.8007788227201]  IrAngle0=[-20.3470720252961 -140.347167299991 99.6528767404244]
      settings: AttributesFormatString=\n  LibrarySourceBlock=sps_lib/Power Grid Elements/Distributed Parameters Line
  MIC-MAN 60 km : spsDistributedParametersLineLib/Distributed Parameters Line  Phases=3  Length=60  Frequency=60  Resistance="[0.01273  0.3864]"  Inductance="[0.9337e-3  4.1264e-3]"  Capacitance=[12.74e-9 7.751e-9]  x1=[-0.000375 3.90848565063247e-09 327054.205336969 -753828.913938461;-0.0003 3.81959620763294e-09 348234.666111732 -744281.641234101;-0.000225 3.7276534378668e-09 369136.753422575 -734139.401173629;-0.00015 3.63273083897744e-09 389743.758460713 -723410.301308568;-7.5e-05 3.53490429063805e-09 410039.208301618 -712102.91831719]  x2=[-0.000375 1.09793181425286e-09 341757.375055572 -724337.843086658;-0.0003 1.04290433287904e-09 362098.228966576 -714386.690108754;-0.000225 9.87043169738486e-10 382149.627093632 -703864.467341261;-0.00015 9.30392979390309e-10 401895.540655875 -692779.586088062;-7.5e-05 8.72999047129898e-10 421320.185072126 -681140.907433628]  x3=[-0.000375 -1.42560259111398e-11 2516.12263919149 -3470.38246360583;-0.0003 -1.50106328260909e-11 2613.22665570694 -3397.86332962471;-0.000225 -1.57532404708311e-11 2708.24169881752 -3322.62799568694;-0.00015 -1.64832552161717e-11 2801.09181495156 -3244.73660376734;-7.5e-05 -1.72000934994947e-11 2891.70278114686 -3164.25141905282]  x4=[-0.000375 2.34755142514101e-11 -263.637973265811 -2074.49907539905;-0.0003 2.41911393543917e-11 -204.88525754252 -2081.12319463934;-0.000225 2.48874264307104e-11 -145.968759679199 -2086.08369584009;-0.00015 2.55638188791307e-11 -86.9355766227876 -2089.37661365253;-7.5e-05 2.62197760018786e-11 -27.8328985965829 -2090.99931576855]  x5=0.000339324940197445  V1=ones(3,3)  V2=ones(3,3)  I1=ones(3,3)  I2=ones(3,3)  nHarmo=1  Measurements=None  Decoupling=on  VsMag0=[670930.718084451 670931.402748886 670930.538861588]  VrMag0=[653943.402704951 653944.061381449 653943.214719902]  VsAngle0=[1.55396261635725 -118.446088813397 121.553886266157]  VrAngle0=[3.35889302260268 -116.641159314998 123.358816875039]  IsMag0=[3504.88423853048 3504.8873913033 3504.88350496928]  IrMag0=[1709.85567574052 1709.85804897088 1709.85543949977]  IsAngle0=[14.0431472467693 -105.956896356636 134.043080810385]  IrAngle0=[-29.1426028746275 -149.142657929214 90.8573007274752]
      settings: AttributesFormatString=\n  LibrarySourceBlock=sps_lib/Power Grid Elements/Distributed Parameters Line
  Regulateurs6 : Subsystem
  Regulateurs7 : Subsystem
  "MIC7a " : PMIOPort  Side=Left
  MIC7b : PMIOPort  Port=2  Side=Left
  MIC7c : PMIOPort  Port=3  Side=Left
  QUE7a : PMIOPort  Port=4  Side=Left
  QUE7b : PMIOPort  Port=5  Side=Left
  QUE7c : PMIOPort  Port=6  Side=Left
  wires:
  Regulateurs6/1(Pm) -> "B_6 CHU-5600 MVA "/1
  Regulateurs6/2(Vf) -> "B_6 CHU-5600 MVA "/2
  "B_6 CHU-5600 MVA "/1 -> Regulateurs6/1(m)
  Regulateurs7/1(Pm) -> B_7 MAN 5000 MVA/1
  Regulateurs7/2(Vf) -> B_7 MAN 5000 MVA/2
  B_7 MAN 5000 MVA/1 -> Regulateurs7/1(m)
  connections:
  "Cs PER "/RConn3 -- MIC-LTD 409 km/LConn3
  "Cs PER "/RConn2 -- MIC-LTD 409 km/LConn2
  "Cs PER "/RConn1 -- MIC-LTD 409 km/LConn1
  Cs BER/RConn3 -- MAN-LEV 3*379km/LConn3
  Cs BER/RConn2 -- MAN-LEV 3*379km/LConn2
  Cs BER/RConn1 -- MAN-LEV 3*379km/LConn1
  Cs ARNS2/RConn3 -- ARN-MAN 2*169km/LConn3
  Cs ARNS2/RConn2 -- ARN-MAN 2*169km/LConn2
  Cs ARNS2/RConn1 -- ARN-MAN 2*169km/LConn1
  CHU-ARN 3*450km/RConn3 -- "Cs MTG+ARNN "/LConn3
  CHU-ARN 3*450km/RConn2 -- "Cs MTG+ARNN "/LConn2
  CHU-ARN 3*450km/RConn1 -- "Cs MTG+ARNN "/LConn1
  Load Flow Bus2/LConn1 -- 5600 MVA 13.8 kV/735 kV1/RConn3 -- CHU-ARN 3*450km/LConn3 -- CHU 330 Mvar/LConn3
  5600 MVA 13.8 kV/735 kV1/RConn2 -- CHU-ARN 3*450km/LConn2 -- CHU 330 Mvar/LConn2
  5600 MVA 13.8 kV/735 kV1/RConn1 -- CHU-ARN 3*450km/LConn1 -- CHU 330 Mvar/LConn1
  "B_6 CHU-5600 MVA "/RConn3 -- Load Flow Bus1/LConn1 -- 5600 MVA 13.8 kV/735 kV1/LConn3 -- 280 MW/LConn3
  5600 MVA 13.8 kV/735 kV1/LConn2 -- "B_6 CHU-5600 MVA "/RConn2 -- 280 MW/LConn2
  5600 MVA 13.8 kV/735 kV1/LConn1 -- "B_6 CHU-5600 MVA "/RConn1 -- 280 MW/LConn1
  "Cs ARNS1 "/RConn1 -- ARN-MIC 180km/LConn1
  "Cs ARNS1 "/RConn2 -- ARN-MIC 180km/LConn2
  "Cs ARNS1 "/RConn3 -- ARN-MIC 180km/LConn3
  "Cs PER "/LConn3 -- Load Flow Bus6/LConn1 -- MIC7c/RConn1 -- MIC-MAN 60 km/LConn3 -- ARN-MIC 180km/RConn3
  "Cs PER "/LConn2 -- MIC7b/RConn1 -- ARN-MIC 180km/RConn2 -- MIC-MAN 60 km/LConn2
  "Cs PER "/LConn1 -- "MIC7a "/RConn1 -- ARN-MIC 180km/RConn1 -- MIC-MAN 60 km/LConn1
  ARN-MAN 2*169km/RConn1 -- MAN7/LConn1
  ARN-MAN 2*169km/RConn2 -- MAN7/LConn2
  ARN-MAN 2*169km/RConn3 -- MAN7/LConn3
  Cs BER/LConn1 -- 5000 MVA 13.8 kV/735 kV2/RConn1 -- MIC-MAN 60 km/RConn1 -- MAN-MIC 1650 Mvar/LConn1 -- MAN7/RConn1
  Cs BER/LConn2 -- 5000 MVA 13.8 kV/735 kV2/RConn2 -- MIC-MAN 60 km/RConn2 -- MAN-MIC 1650 Mvar/LConn2 -- MAN7/RConn2
  Cs BER/LConn3 -- Load Flow Bus5/LConn1 -- 5000 MVA 13.8 kV/735 kV2/RConn3 -- MIC-MAN 60 km/RConn3 -- MAN-MIC 1650 Mvar/LConn3 -- MAN7/RConn3
  B_7 MAN 5000 MVA/RConn1 -- 5000 MVA 13.8 kV/735 kV2/LConn1 -- 250 MW/LConn1
  B_7 MAN 5000 MVA/RConn2 -- 5000 MVA 13.8 kV/735 kV2/LConn2 -- 250 MW/LConn2
  B_7 MAN 5000 MVA/RConn3 -- 5000 MVA 13.8 kV/735 kV2/LConn3 -- Load Flow Bus3/LConn1 -- 250 MW/LConn3
  MIC-LTD 409 km/RConn2 -- MAN-LEV 3*379km/RConn2 -- QUE7b/RConn1
  Cs ARNS2/LConn1 -- ARN 990 Mvar/LConn1 -- "Cs MTG+ARNN "/RConn1 -- "Cs ARNS1 "/LConn1
  Cs ARNS2/LConn2 -- ARN 990 Mvar/LConn2 -- "Cs MTG+ARNN "/RConn2 -- "Cs ARNS1 "/LConn2
  Cs ARNS2/LConn3 -- Load Flow Bus4/LConn1 -- "Cs ARNS1 "/LConn3 -- ARN 990 Mvar/LConn3 -- "Cs MTG+ARNN "/RConn3
  MIC-LTD 409 km/RConn1 -- QUE7a/RConn1 -- MAN-LEV 3*379km/RConn1
  MIC-LTD 409 km/RConn3 -- QUE7c/RConn1 -- MAN-LEV 3*379km/RConn3
